simulink model "state_double_UnitDelay"  (R2014a)
settings: Solver=FixedStepDiscrete  StartTime=0.0  StopTime=10.0  FixedStep=0.1  RelTol=1e-3
settings Model: Creator=yoshi12  LastModifiedBy=yoshi12

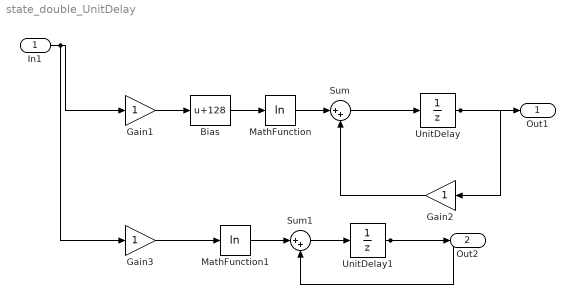
== system state_double_UnitDelay ==
  In1 : Inport
  Bias : Bias  Bias=128
  Gain1 : Gain
  Gain2 : Gain
  Gain3 : Gain
  MathFunction : Math  Operator=log  SaturateOnIntegerOverflow=on
  MathFunction1 : Math  Operator=log  SaturateOnIntegerOverflow=on
  Sum : Sum  Inputs=|++
  Sum1 : Sum  Inputs=|++
  UnitDelay : UnitDelay  SampleTime=-1
  UnitDelay1 : UnitDelay  SampleTime=-1
  Out1 : Outport
  Out2 : Outport  Port=2
  wires:
  Sum/1 -> UnitDelay/1
  UnitDelay/1 -> Gain2/1, Out1/1
  In1/1 -> Gain3/1, Gain1/1
  Gain1/1 -> Bias/1
  Bias/1 -> MathFunction/1
  Gain2/1 -> Sum/2
  MathFunction/1 -> Sum/1
  Gain3/1 -> MathFunction1/1
  MathFunction1/1 -> Sum1/1
  UnitDelay1/1 -> Sum1/2, Out2/1
  Sum1/1 -> UnitDelay1/1
